simulink model "Boost_Converter_Modelling"  (R2015a)
settings: Solver=ode45  StartTime=0.0  StopTime=0.1  RelTol=1e-3
values from neighbouring files (symbols this model uses):
  C = 45e-06    (= 4.5e-05)    [BOOST_CONVERTER_SCRIPT.m]
  D = 0.4    [BOOST_CONVERTER_SCRIPT.m]
  fs = 51e03    (= 51000)    [BOOST_CONVERTER_SCRIPT.m]
  L = 255e-06    (= 0.000255)    [BOOST_CONVERTER_SCRIPT.m]
  R = 26    [BOOST_CONVERTER_SCRIPT.m]
  Vin = 132    [BOOST_CONVERTER_SCRIPT.m]
settings Model: Creator=Koustubh  LastModifiedBy=Koustubh

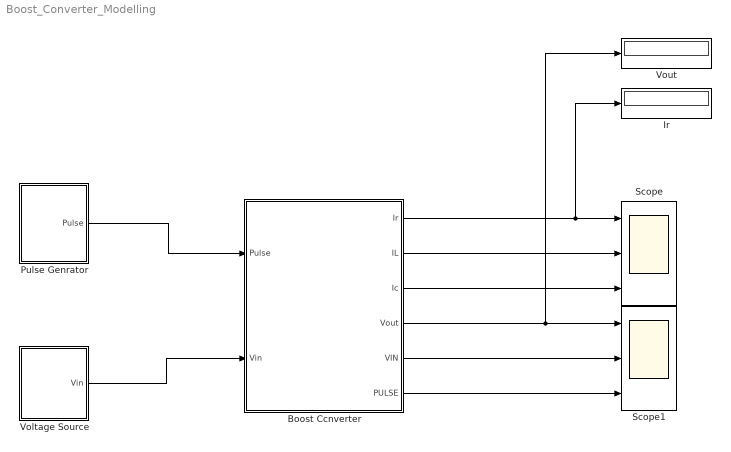
== system Boost_Converter_Modelling ==
  Boost Ccnverter : Subsystem
  Ir : Display
  Pulse Genrator : Subsystem
  Scope : Scope  NumInputPorts=3
      settings: YMin=-5~-5~-5  YMax=5~5~5
  Scope1 : Scope  NumInputPorts=3
      settings: YMin=-5~-5~-5  YMax=5~5~5
  Voltage Source : Subsystem
  Vout : Display
  wires:
  Pulse Genrator/1(Pulse) -> Boost Ccnverter/1(Pulse)
  Voltage Source/1(Vin) -> Boost Ccnverter/2(Vin)
  Boost Ccnverter/2(IL) -> Scope/2
  Boost Ccnverter/1(Ir) -> Ir/1, Scope/1
  Boost Ccnverter/3(Ic) -> Scope/3
  Boost Ccnverter/4(Vout) -> Vout/1, Scope1/1
  Boost Ccnverter/5(VIN) -> Scope1/2
  Boost Ccnverter/6(PULSE) -> Scope1/3

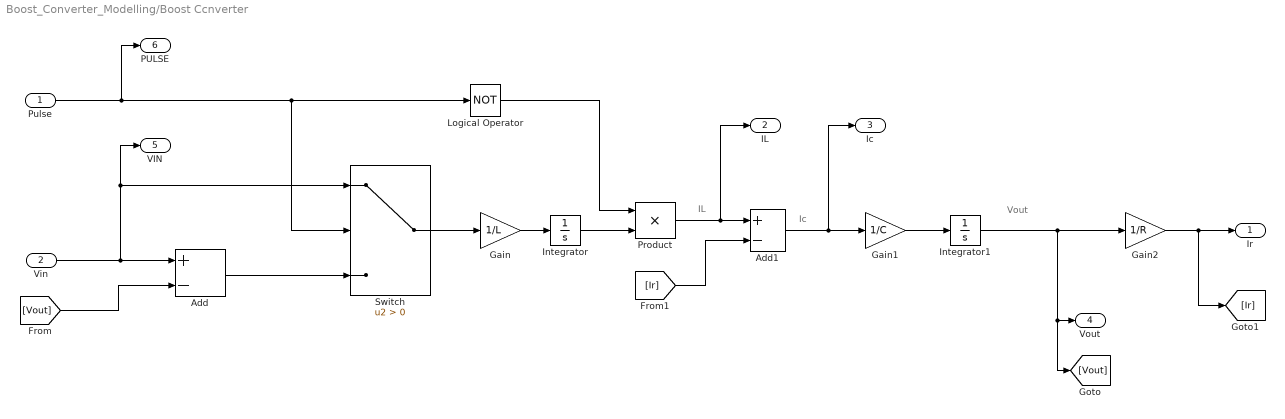
== system Boost_Converter_Modelling/Boost Ccnverter ==
  note: Vout
  note: Ic
  note: IL
  Pulse : Inport
  Vin : Inport  Port=2
  Add : Sum  Inputs=+-
  Add1 : Sum  Inputs=+-
  Gain : Gain  Gain=1/L
  Gain1 : Gain  Gain=1/C
  Gain2 : Gain  Gain=1/R
  Integrator : Integrator
  Integrator1 : Integrator
  Logical Operator : Logic  Operator=NOT  AllPortsSameDT=off  OutDataTypeStr=boolean
  Product : Product
  Switch : Switch  Criteria=u2 > Threshold
  Ir : Outport
  IL : Outport  Port=2
  Ic : Outport  Port=3
  Vout : Outport  Port=4
  VIN : Outport  Port=5
  PULSE : Outport  Port=6
  wires:
  Vin/1 -> VIN/1, Switch/1, Add/1
  Add/1 -> Switch/3
  [Vout] -> Add/2
  Pulse/1 -> PULSE/1, Logical Operator/1, Switch/2
  Switch/1 -> Gain/1
  Gain/1 -> Integrator/1
  Integrator/1 -> Product/2
  Logical Operator/1 -> Product/1
  Product/1 -> IL/1, Add1/1
  [Ir] -> Add1/2
  Add1/1 -> Ic/1, Gain1/1
  Gain1/1 -> Integrator1/1
  Integrator1/1 -> Vout/1, [Vout], Gain2/1
  Gain2/1 -> [Ir], Ir/1

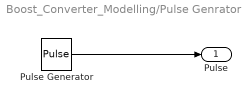
== system Boost_Converter_Modelling/Pulse Genrator ==
  Pulse Generator : DiscretePulseGenerator  PulseType=Time based  Period=1/fs  PulseWidth=D*100
  Pulse : Outport
  wires:
  Pulse Generator/1 -> Pulse/1

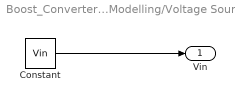
== system Boost_Converter_Modelling/Voltage Source ==
  Constant : Constant  Value=Vin
  Vin : Outport
  wires:
  Constant/1 -> Vin/1
